simulink model "model3part1"  (R2018b)
settings: Solver=VariableStepAuto  StartTime=0.0  StopTime=10.0  RelTol=1e-3
values from neighbouring files (symbols this model uses):
  A = amp(i)    [script3.m]
  g21 = [1]    [script3.m]
  g22 = [1 0.1 1]    [script3.m]
  gd1 = g21    [script3.m]
  gd2 = g22    [script3.m]
  gg1 = [0.4 0]    [script3.m]
  gg2 = [0.4 1]    [script3.m]
  gp1 = [1 0]    [script3.m]
  gp2 = [1 2 1]    [script3.m]
  om = omega(i)    [script3.m]
  PHI = phi(i)    [script3.m]
settings Model: Creator=Joanna  LastModifiedBy=Joanna

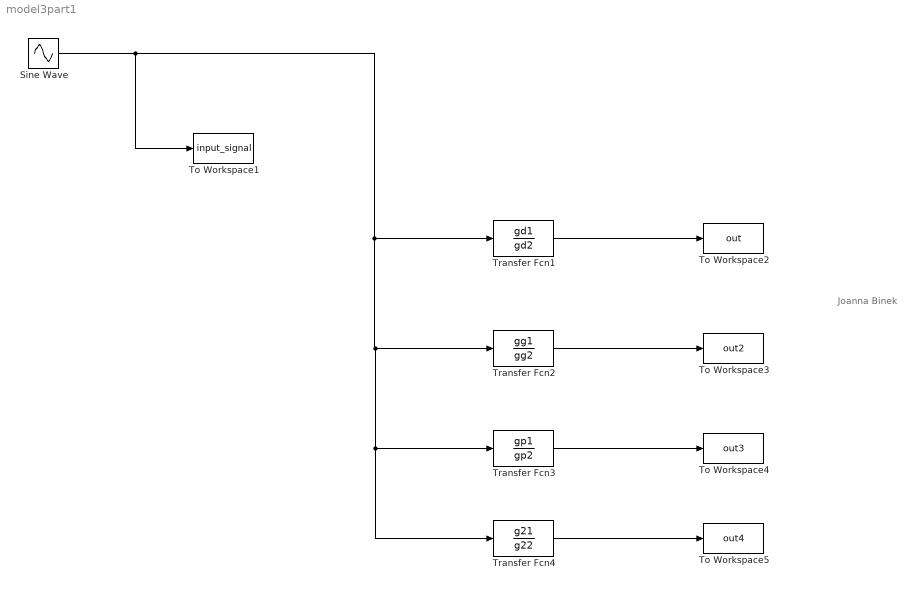
== system model3part1 ==
  note: Joanna Binek
  Sine Wave : Sin  Amplitude=A  Frequency=om  Phase=PHI  SampleTime=0
  To Workspace1 : ToWorkspace  VariableName=input_signal  SampleTime=-1
  To Workspace2 : ToWorkspace  VariableName=out  SampleTime=-1
  To Workspace3 : ToWorkspace  VariableName=out2  SampleTime=-1
  To Workspace4 : ToWorkspace  VariableName=out3  SampleTime=-1
  To Workspace5 : ToWorkspace  VariableName=out4  SampleTime=-1
  Transfer Fcn1 : TransferFcn  Numerator=gd1  Denominator=gd2
  Transfer Fcn2 : TransferFcn  Numerator=gg1  Denominator=gg2
  Transfer Fcn3 : TransferFcn  Numerator=gp1  Denominator=gp2
  Transfer Fcn4 : TransferFcn  Numerator=g21  Denominator=g22
  wires:
  Transfer Fcn4/1 -> To Workspace5/1
  Transfer Fcn3/1 -> To Workspace4/1
  Transfer Fcn1/1 -> To Workspace2/1
  Transfer Fcn2/1 -> To Workspace3/1
  Sine Wave/1 -> Transfer Fcn1/1, Transfer Fcn2/1, Transfer Fcn4/1, Transfer Fcn3/1, To Workspace1/1
